simulink library "TBONE"  (R2021b)
settings: Solver=VariableStepAuto  StartTime=0.0  StopTime=10.0  RelTol=1e-3
undefined symbols (not defined in the file): FlowStartVol, Fluid, Lib_Vol_FlowStart_TMATS
libraries: Lib_Vol_FlowChar_TMATS x4, Lib_Vol_Pipe_TMATS x4, Lib_Vol_Volume_TMATS x4, Lib_Vol_Valve_TMATS x4, Lib_Vol_PropLookup_TMATS x1, $bdroot x1
settings Model: Creator=ashwi  LastModifiedBy=ashwi

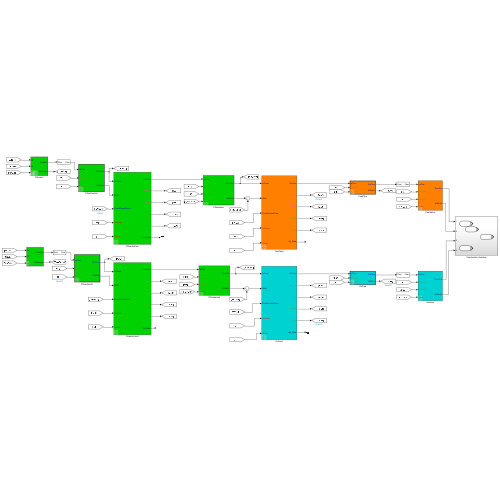
[thumbnail: Simulink's stored preview of the top-level diagram]
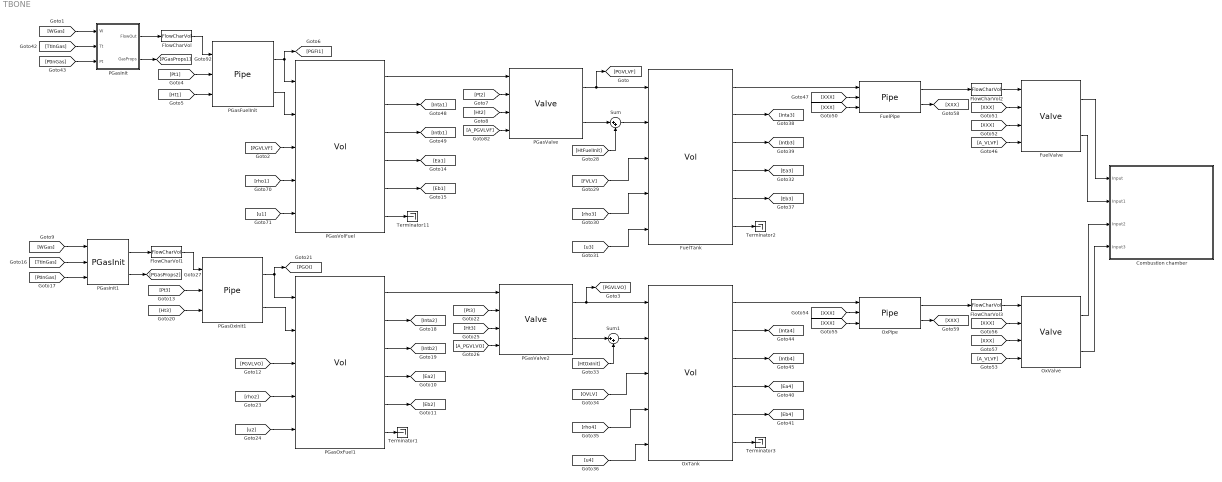
== system TBONE ==
  Combustion chamber : Subsystem
  FlowCharVol{,1..3} (4 alike) : Lib_Vol_FlowChar_TMATS/FlowCharVol  SystemSampleTime=-1  VariantActivationTime=update diagram  Latency=0  AutoFrameSizeCalculation=off
  FuelPipe : Lib_Vol_Pipe_TMATS/Pipe  Diameter=1  Length=24  htVec_M=Fluid.Vec.ht  PtVec_M=Fluid.Vec.Pt  TtArray_M=Fluid.Array.Tt  rhoArray_M=Fluid.Array.rho
  FuelTank : Lib_Vol_Volume_TMATS/Vol  volume_M=1  htVec_M=Fluid.Vec.ht  PtVec_M=Fluid.Vec.Pt  TtArray_M=Fluid.Array.Tt  uArray_M=Fluid.Array.u  rhoArray_M=Fluid.Array.rho
  FuelValve : Lib_Vol_Valve_TMATS/Valve  Cd_M=0.6  htVec_M=Fluid.Vec.ht  PtVec_M=Fluid.Vec.Pt  TtArray_M=Fluid.Array.Tt  rhoArray_M=Fluid.Array.rho
  OxPipe : Lib_Vol_Pipe_TMATS/Pipe  Diameter=1  Length=24  htVec_M=Fluid.Vec.ht  PtVec_M=Fluid.Vec.Pt  TtArray_M=Fluid.Array.Tt  rhoArray_M=Fluid.Array.rho
  OxTank : Lib_Vol_Volume_TMATS/Vol  volume_M=1  htVec_M=Fluid.Vec.ht  PtVec_M=Fluid.Vec.Pt  TtArray_M=Fluid.Array.Tt  uArray_M=Fluid.Array.u  rhoArray_M=Fluid.Array.rho
  OxValve : Lib_Vol_Valve_TMATS/Valve  Cd_M=0.6  htVec_M=Fluid.Vec.ht  PtVec_M=Fluid.Vec.Pt  TtArray_M=Fluid.Array.Tt  rhoArray_M=Fluid.Array.rho
  PGasFuelInit : Lib_Vol_Pipe_TMATS/Pipe  Diameter=1  Length=24  htVec_M=Fluid.Vec.ht  PtVec_M=Fluid.Vec.Pt  TtArray_M=Fluid.Array.Tt  rhoArray_M=Fluid.Array.rho
  PGasInit : Subsystem  AncestorBlock=Lib_Vol_FlowStart_TMATS/FlowStartVol  mask(T-MATS: FlowStart Library Block){TtVec_M=Fluid.Vec.Tt, PtVec_M=Fluid.Vec.Pt, htVec_M=Fluid.Vec.ht, sVec_M=Fluid.Vec.s, htArray_M=Fluid.Array.ht, TtArray_M=Fluid.Array.Tt, sArray_M=Fluid.Array.s, rhoArray_M=Fluid.Array.rho, muArray_M=Fluid.Array.mu, CpArray_M=Fluid.Array.Cp, CvArray_M=Fluid.Array.Cv, CvArray_M_copy=Fluid.Array.u, Rval_M=Fluid.Array.R}
      mask prompts: TtVec_M "TtVec_M - Temperature vector"; PtVec_M "PtVec_M - Pressure vector"; htVec_M "htVec_M - Enthalpy vector"; sVec_M "sVec_M - Entropy vector"; htArray_M "htArray_M - Enthalpy Array f(Tt,Pt)"; TtArray_M "TtArray_M - Temperature Array f(ht,Pt)"; sArray_M "sArray_M - Entropy Array f(ht,Pt)"; rhoArray_M "rhoArray_M - Density Array f(ht,Pt)"; muArray_M "muArray_M - Viscosity Array f(ht,Pt)"; CpArray_M "CpArray_M - Pressure specific heat Array f(ht,Pt)"; CvArray_M "CvArray_M - Volume specific heat Array f(ht,Pt)"; CvArray_M_copy "uArray_M - Internal energy Array f(ht,Pt)"; Rval_M "Rval_M - R value"
      mask help: This block simulates the initialization of fluid properties through a lookup table based on total pressure and temperature.
      mask Help: web(which('Vol_TMATS FlowStart.html'),'-helpbrowser')
  PGasInit1 : $bdroot/PGasInit  TtVec_M=Fluid.Vec.Tt  PtVec_M=Fluid.Vec.Pt  htVec_M=Fluid.Vec.ht  sVec_M=Fluid.Vec.s  htArray_M=Fluid.Array.ht  TtArray_M=Fluid.Array.Tt  sArray_M=Fluid.Array.s  rhoArray_M=Fluid.Array.rho  muArray_M=Fluid.Array.mu  CpArray_M=Fluid.Array.Cp  CvArray_M=Fluid.Array.Cv  CvArray_M_copy=Fluid.Array.u  Rval_M=Fluid.Array.R
  PGasOxFuel1 : Lib_Vol_Volume_TMATS/Vol  volume_M=1  htVec_M=Fluid.Vec.ht  PtVec_M=Fluid.Vec.Pt  TtArray_M=Fluid.Array.Tt  uArray_M=Fluid.Array.u  rhoArray_M=Fluid.Array.rho
  PGasOxInit1 : Lib_Vol_Pipe_TMATS/Pipe  Diameter=1  Length=24  htVec_M=Fluid.Vec.ht  PtVec_M=Fluid.Vec.Pt  TtArray_M=Fluid.Array.Tt  rhoArray_M=Fluid.Array.rho
  PGasValve : Lib_Vol_Valve_TMATS/Valve  Cd_M=3.4641  htVec_M=Fluid.Vec.ht  PtVec_M=Fluid.Vec.Pt  TtArray_M=Fluid.Array.Tt  rhoArray_M=Fluid.Array.rho
  PGasValve2 : Lib_Vol_Valve_TMATS/Valve  Cd_M=3.4641  htVec_M=Fluid.Vec.ht  PtVec_M=Fluid.Vec.Pt  TtArray_M=Fluid.Array.Tt  rhoArray_M=Fluid.Array.rho
  PGasVolFuel : Lib_Vol_Volume_TMATS/Vol  volume_M=1  htVec_M=Fluid.Vec.ht  PtVec_M=Fluid.Vec.Pt  TtArray_M=Fluid.Array.Tt  uArray_M=Fluid.Array.u  rhoArray_M=Fluid.Array.rho
  Sum : Sum  Inputs=|++
  Sum1 : Sum  Inputs=|++
  Terminator{1..3,11} (4 alike) : Terminator
  wires:
  PGasInit/1(FlowOut) -> FlowCharVol/1
  FlowCharVol/1 -> PGasFuelInit/1
  PGasFuelInit/1 -> PGasVolFuel/1, [PGFI1]
  PGasFuelInit/2 -> PGasVolFuel/2
  [TtInGas] -> PGasInit/2("Tt ")
  [PtInGas] -> PGasInit/3(Pt)
  [WGas] -> PGasInit/1(W)
  PGasInit/2(GasProps) -> [PGasProps1]
  [Pt1] -> PGasFuelInit/2
  [Ht1] -> PGasFuelInit/3
  [Ht2] -> PGasValve/3
  PGasValve/1 -> [PGVLVF], FuelTank/1
  [Pt2] -> PGasValve/2
  [A_PGVLVF] -> PGasValve/4
  PGasVolFuel/6 -> Terminator11/1
  PGasVolFuel/2 -> [Inta1]
  PGasVolFuel/3 -> [Intb1]
  PGasVolFuel/4 -> [Ea1]
  PGasVolFuel/5 -> [Eb1]
  PGasVolFuel/1 -> PGasValve/1
  [u1] -> PGasVolFuel/5
  [rho1] -> PGasVolFuel/4
  [PGVLVF] -> PGasVolFuel/3
  [WGas] -> PGasInit1/1
  [u2] -> PGasOxFuel1/5
  [TtInGas] -> PGasInit1/2
  PGasOxFuel1/6 -> Terminator1/1
  PGasOxFuel1/5 -> [Eb2]
  [Pt3] -> PGasOxInit1/2
  PGasOxFuel1/2 -> [Inta2]
  PGasOxFuel1/4 -> [Ea2]
  [Ht3] -> PGasOxInit1/3
  PGasInit1/1 -> FlowCharVol1/1
  [rho2] -> PGasOxFuel1/4
  PGasOxFuel1/3 -> [Intb2]
  PGasInit1/2 -> [PGasProps2]
  [PtInGas] -> PGasInit1/3
  PGasOxInit1/1 -> PGasOxFuel1/1, [PGOI]
  FlowCharVol1/1 -> PGasOxInit1/1
  [Pt3] -> PGasValve2/2
  PGasOxFuel1/1 -> PGasValve2/1
  PGasValve2/1 -> OxTank/1, [PGVLVO]
  [PGVLVO] -> PGasOxFuel1/3
  [Ht3] -> PGasValve2/3
  [A_PGVLVO] -> PGasValve2/4
  PGasOxInit1/2 -> PGasOxFuel1/2
  PGasValve/2 -> Sum/1
  Sum/1 -> FuelTank/2
  [HtFuelInit] -> Sum/2
  [rho3] -> FuelTank/4
  [u3] -> FuelTank/5
  [FVLV] -> FuelTank/3
  [rho4] -> OxTank/4
  Sum1/1 -> OxTank/2
  [HtOxInit] -> Sum1/2
  [u4] -> OxTank/5
  [OVLV] -> OxTank/3
  PGasValve2/2 -> Sum1/1
  FuelTank/4 -> [Ea3]
  FuelTank/3 -> [Intb3]
  FuelTank/2 -> [Inta3]
  FuelTank/5 -> [Eb3]
  FuelTank/6 -> Terminator2/1
  OxTank/5 -> [Eb4]
  OxTank/3 -> [Intb4]
  OxTank/4 -> [Ea4]
  OxTank/6 -> Terminator3/1
  OxTank/2 -> [Inta4]
  FuelTank/1 -> FuelPipe/1
  FuelPipe/1 -> FlowCharVol2/1
  FlowCharVol2/1 -> FuelValve/1
  [A_VLVF] -> FuelValve/4
  [XXX] -> FuelPipe/2
  [XXX] -> FuelPipe/3
  [XXX] -> FuelValve/2
  [XXX] -> FuelValve/3
  [XXX] -> OxValve/2
  FlowCharVol3/1 -> OxValve/1
  [XXX] -> OxPipe/2
  OxPipe/1 -> FlowCharVol3/1
  OxTank/1 -> OxPipe/1
  [XXX] -> OxValve/3
  [A_VLVF] -> OxValve/4
  [XXX] -> OxPipe/3
  FuelValve/1 -> Combustion chamber/1(Input)
  FuelValve/2 -> Combustion chamber/2(Input1)
  OxValve/1 -> Combustion chamber/3(Input2)
  OxValve/2 -> Combustion chamber/4(Input3)
  FuelPipe/2 -> [XXX]
  OxPipe/2 -> [XXX]

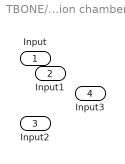
== system TBONE/Combustion chamber ==
  Input : Inport
  Input1 : Inport  Port=2
  Input2 : Inport  Port=3
  Input3 : Inport  Port=4

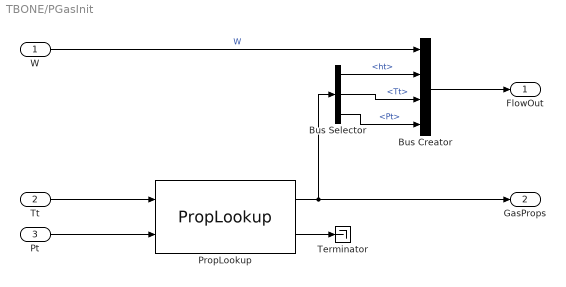
== system TBONE/PGasInit ==
  W : Inport
  "Tt " : Inport  Port=2
  Pt : Inport  Port=3
  Bus Creator : BusCreator  Inputs=4
  Bus Selector : BusSelector  OutputSignals=ht,Tt,Pt
  PropLookup : Lib_Vol_PropLookup_TMATS/PropLookup  case_M='Tt'  propg_M=0  htg_M=0  htVec_M=htVec_M  PtVec_M=PtVec_M  TtVec_M=TtVec_M  sVec_M=sVec_M  htArray_M=htArray_M  rhoArray_M=rhoArray_M  uArray_M=ones(length(htVec_M), length(PtVec_M))'  sArray_M=sArray_M  muArray_M=muArray_M  ThArray_M=TtArray_M  CvArray_M=CvArray_M  CpArray_M=CpArray_M  kArray_M=ones(length(htVec_M), length(PtVec_M))'  TsArray_M=ones(length(sVec_M), length(PtVec_M))'  hsArray_M=ones(length(sVec_M), length(PtVec_M))'  Rval_M=Rval_M
  Terminator : Terminator
  FlowOut : Outport
  GasProps : Outport  Port=2
  wires:
  Bus Creator/1 -> FlowOut/1
  W/1 -> Bus Creator/1  "W"
  Pt/1 -> PropLookup/2
  "Tt "/1 -> PropLookup/1
  PropLookup/2 -> Terminator/1
  PropLookup/1 -> GasProps/1, Bus Selector/1
  Bus Selector/3 -> Bus Creator/4  "<Pt>"
  Bus Selector/2 -> Bus Creator/3  "<Tt>"
  Bus Selector/1 -> Bus Creator/2  "<ht>"
